simulink model "NeuralNetUnitLDC"  (R2018b)
settings: Solver=FixedStepAuto  StartTime=0.0  StopTime=20  FixedStep=0.05  RelTol=1e-3
values from neighbouring files (symbols this model uses):
  B = 0.2    [SampleDCmachineParameters.m]
  b = 0.08    [SampleDCmachineParameters.m]
  l = 0.6    [SampleDCmachineParameters.m]
  m = 0.1    [SampleDCmachineParameters.m]
  R = 5    [SampleDCmachineParameters.m]
settings Model: Creator=Therecia  LastModifiedBy=Tyson
settings DebuggingCC: InheritedTsInSrcMsg=none  LibraryContextMissingDiagnostic=none
settings SFSimCC: SimUseLocalCustomCode=off
settings RTWCC: RTWUseLocalCustomCode=off
settings CodeAppCC: StateflowObjectComments=on

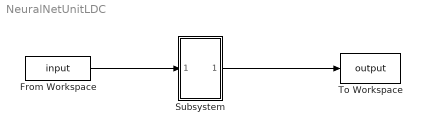
== system NeuralNetUnitLDC ==
  From Workspace : FromWorkspace  VariableName=input
  Subsystem : Subsystem
      mask DialogControl Control2 Prompt: BlackBox
  To Workspace : ToWorkspace  VariableName=output  SaveFormat=Timeseries  SampleTime=-1
  wires:
  From Workspace/1 -> Subsystem/1(In1)
  Subsystem/1(Out1) -> To Workspace/1

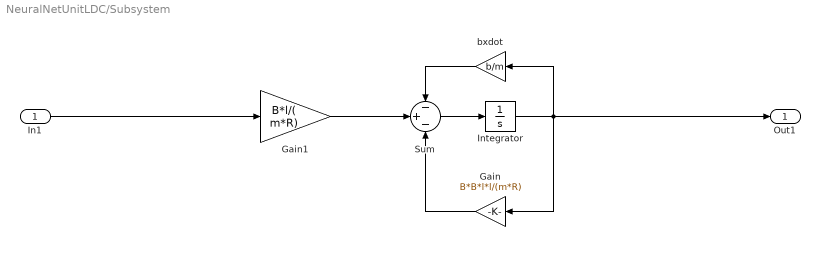
== system NeuralNetUnitLDC/Subsystem ==
  In1 : Inport
  Gain : Gain  Gain=B*B*l*l/(m*R)
  Gain1 : Gain  Gain=B*l/( m*R)
  Integrator : Integrator
  Sum : Sum  Inputs=-+-
  bxdot : Gain  Gain=b/m
  Out1 : Outport
  wires:
  In1/1 -> Gain1/1
  Sum/1 -> Integrator/1
  Gain/1 -> Sum/3
  Integrator/1 -> Out1/1, bxdot/1, Gain/1
  Gain1/1 -> Sum/2
  bxdot/1 -> Sum/1
